simulink model "SIM_model_model_befMERGE"  (R2026a)
settings: Solver=ode4  StopTime=10  FixedStep=0.01
InitFcn:
  | initFcn;
undefined symbols (not defined in the file or in its folder): rocket
libraries: aerolibasang x2, aerolibanim x1, simulink x1, aerolibfltsims x1, aerolibatmos2 x1, aerolibadyn x1
settings Model: Creator=carlos  LastModifiedBy=carlos

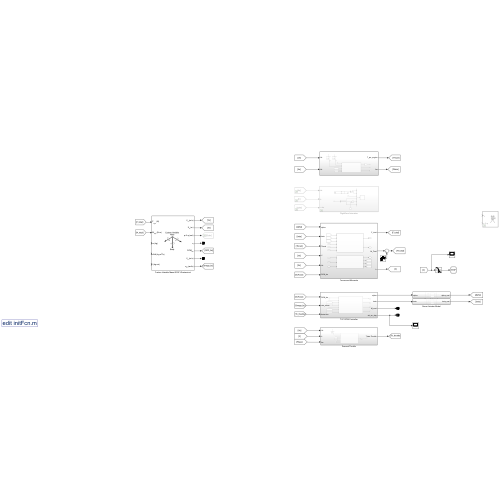
[thumbnail: Simulink's stored preview of the top-level diagram]
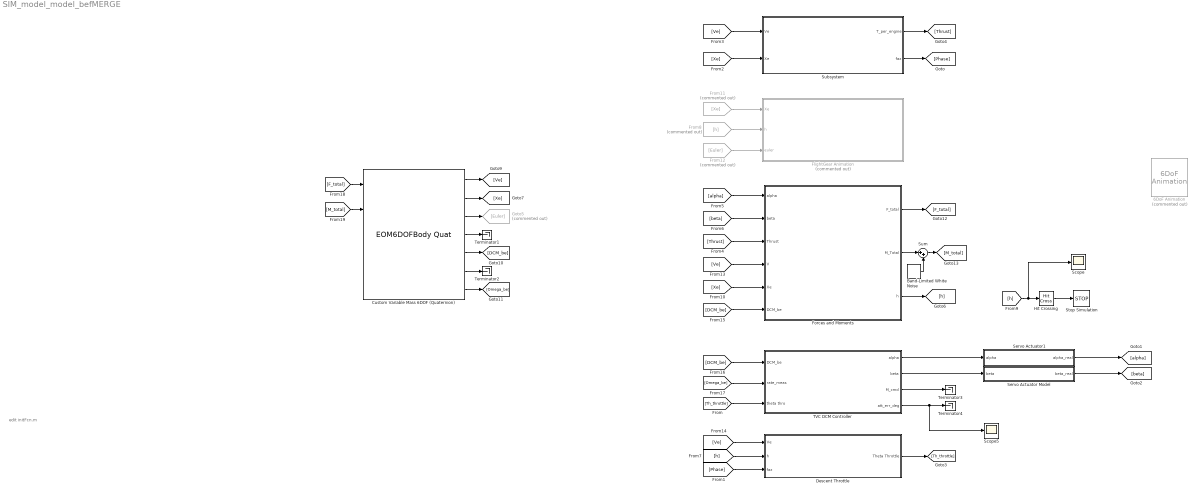
== system SIM_model_model_befMERGE ==
  note: edit initFcn.m
  6DoF Animation : aerolibanim/6DoF Animation  Commented=on  u1=[-100 100 -100 100 0 3000]  u2=0.1  u3=200  u4=[0 0 0]  u5=Fixed position  u6=[7500 7500 -3150]  u7=10  u8=on
  Band-Limited White Noise : simulink/Sources/Band-Limited White Noise  Cov=4e-6  Ts=0.01  seed=[23341 23342 23343]
  Custom Variable Mass 6DOF (Quaternion) : EOM6DOFBodyQuat  mtype=Custom Variable  eul_0=[0 deg2rad(90) 0]
  Descent Throttle : Subsystem
  FlightGear Animation : Subsystem  Commented=on
  Forces and Moments : Subsystem
  From11 : From  Commented=on  GotoTag=Xe
  From12 : From  Commented=on  GotoTag=Euler
  From8 : From  Commented=on  GotoTag=h
  Goto5 : Goto  Commented=on  GotoTag=Euler
  Hit Crossing : HitCross  HitCrossingDirection=falling
  Scope : Scope
      settings: ActiveDisplayYMinimum=-1.94208  ActiveDisplayYMaximum=17.47869
  Scope5 : Scope
      settings: ActiveDisplayYMinimum=-20.36974  ActiveDisplayYMaximum=7.70273  DataLoggingVariableName=ScopeData7
  Servo Actuator Model : Subsystem
  Servo Actuator1 : Subsystem
  Stop Simulation : Stop
  Subsystem : Subsystem
  Sum : Sum  Inputs=|++
  TVC DCM Controller : Subsystem
  Terminator{1..4} (4 alike) : Terminator
  wires:
  Sum/1 -> [M_total]
  Forces and Moments/2(M_Total) -> Sum/1
  Band-Limited White Noise/1 -> Sum/2
  [alpha] -> Forces and Moments/1(alpha)
  [DCM_be] -> Forces and Moments/6(DCM_be)
  [beta] -> Forces and Moments/2(beta)
  [Xe] -> Forces and Moments/5(Xe)
  [Thrust] -> Forces and Moments/3(Thrust)
  Forces and Moments/3(h) -> [h]
  Forces and Moments/1(F_total) -> [F_total]
  [Ve] -> Forces and Moments/4(V)
  Custom Variable Mass 6DOF (Quaternion)/1 -> [Ve]
  Custom Variable Mass 6DOF (Quaternion)/2 -> [Xe]
  Custom Variable Mass 6DOF (Quaternion)/5 -> [DCM_be]
  Custom Variable Mass 6DOF (Quaternion)/7 -> [Omega_be]
  Custom Variable Mass 6DOF (Quaternion)/6 -> Terminator2/1
  Custom Variable Mass 6DOF (Quaternion)/4 -> Terminator1/1
  [M_total] -> Custom Variable Mass 6DOF (Quaternion)/2
  [F_total] -> Custom Variable Mass 6DOF (Quaternion)/1
  Custom Variable Mass 6DOF (Quaternion)/3 -> Goto5/1
  [h] -> Descent Throttle/2(h)
  TVC DCM Controller/4(att_err_deg) -> Scope5/1, Terminator4/1
  [DCM_be] -> TVC DCM Controller/1(DCM_be)
  [Th_throttle] -> TVC DCM Controller/3(theta thro)
  [Phase] -> Descent Throttle/3(faz)
  [Omega_be] -> TVC DCM Controller/2(rate_meas)
  Descent Throttle/1(Theta Throttle) -> [Th_throttle]
  [Ve] -> Descent Throttle/1(Ve)
  Servo Actuator1/1(alpha_real) -> [alpha]
  TVC DCM Controller/3(M_cmd) -> Terminator3/1
  TVC DCM Controller/2(beta) -> Servo Actuator Model/1(beta)
  Servo Actuator Model/1(beta_real) -> [beta]
  TVC DCM Controller/1(alpha) -> Servo Actuator1/1(alpha)
  Subsystem/2(faz) -> [Phase]
  Subsystem/1(T_per_engine) -> [Thrust]
  [Ve] -> Subsystem/1(Ve)
  [Xe] -> Subsystem/2(Xe)
  From8/1 -> FlightGear Animation/2(h)
  From12/1 -> FlightGear Animation/3(euler)
  From11/1 -> FlightGear Animation/1(Xe)
  [h] -> Scope/1, Hit Crossing/1
  Hit Crossing/1 -> Stop Simulation/1

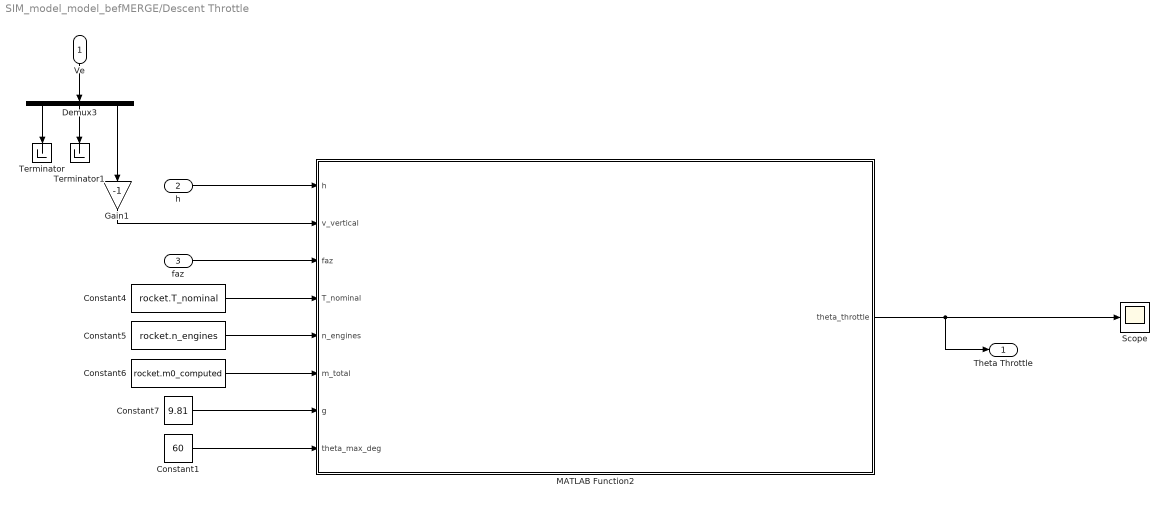
== system SIM_model_model_befMERGE/Descent Throttle ==
  Ve : Inport
  h : Inport  Port=2
  faz : Inport  Port=3
  Constant1 : Constant  Value=60
  Constant4 : Constant  Value=rocket.T_nominal
  Constant5 : Constant  Value=rocket.n_engines
  Constant6 : Constant  Value=rocket.m0_computed
  Constant7 : Constant  Value=9.81
  Demux3 : Demux  Outputs=3
  Gain1 : Gain  Gain=-1
  MATLAB Function2 : MATLAB Function  TreatAsAtomicUnit=on
  Scope : Scope
      settings: ActiveDisplayYMinimum=-0.1309  ActiveDisplayYMaximum=1.1781  DataLoggingVariableName=ScopeData6
  Terminator : Terminator
  Terminator1 : Terminator
  Theta Throttle : Outport
  wires:
  Ve/1 -> Demux3/1
  Demux3/3 -> Gain1/1
  Demux3/2 -> Terminator1/1
  Demux3/1 -> Terminator/1
  h/1 -> MATLAB Function2/1(h)
  Gain1/1 -> MATLAB Function2/2(v_vertical)
  Constant7/1 -> MATLAB Function2/7(g)
  Constant5/1 -> MATLAB Function2/5(n_engines)
  Constant6/1 -> MATLAB Function2/6(m_total)
  Constant4/1 -> MATLAB Function2/4(T_nominal)
  MATLAB Function2/1(theta_throttle) -> Theta Throttle/1, Scope/1
  faz/1 -> MATLAB Function2/3(faz)
  Constant1/1 -> MATLAB Function2/8(theta_max_deg)

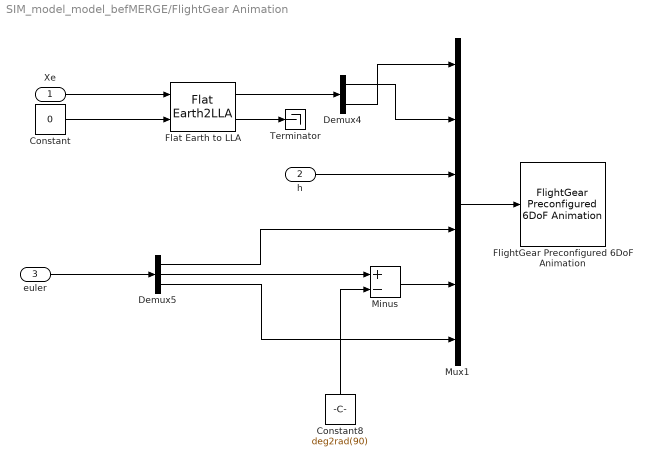
== system SIM_model_model_befMERGE/FlightGear Animation ==
  Xe : Inport
  h : Inport  Port=2
  euler : Inport  Port=3
  Constant : Constant  Value=0
  Constant8 : Constant  Value=deg2rad(90)
  Demux4 : Demux  Outputs=2
  Demux5 : Demux  Outputs=3
  Flat Earth to LLA : FlatEarth2LLA  R=6378137  LL0=[37.61889 -122.37500]
  FlightGear Preconfigured 6DoF Animation : aerolibfltsims/FlightGear Preconfigured 6DoF Animation  xFlightGearVersion=v2019.1  DestinationIpAddress=127.0.0.1  DestinationPort=5502  SampleTime=1/30  packetVersion=24
  Minus : Sum  Inputs=+-
  Mux1 : Mux  Inputs=6
  Terminator : Terminator
  wires:
  Constant/1 -> Flat Earth to LLA/2
  Demux4/1 -> Mux1/2
  Constant8/1 -> Minus/2
  Demux5/2 -> Minus/1
  Minus/1 -> Mux1/5
  Demux5/1 -> Mux1/4
  Demux5/3 -> Mux1/6
  Mux1/1 -> FlightGear Preconfigured 6DoF Animation/1
  Demux4/2 -> Mux1/1
  Flat Earth to LLA/1 -> Demux4/1
  Flat Earth to LLA/2 -> Terminator/1
  euler/1 -> Demux5/1
  h/1 -> Mux1/3
  Xe/1 -> Flat Earth to LLA/1

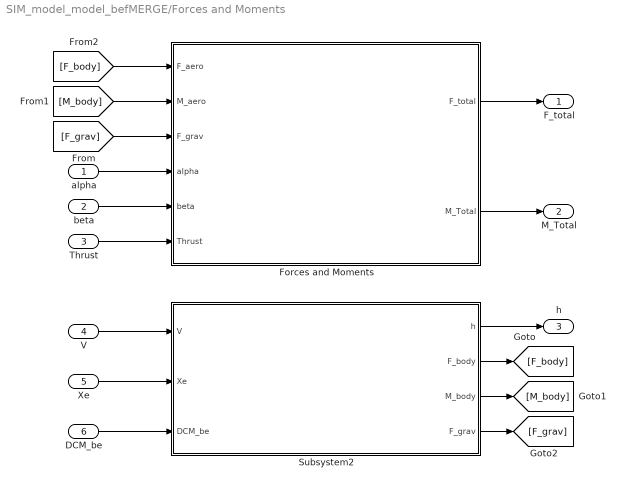
== system SIM_model_model_befMERGE/Forces and Moments ==
  alpha : Inport
  beta : Inport  Port=2
  Thrust : Inport  Port=3
  V : Inport  Port=4
  Xe : Inport  Port=5
  DCM_be : Inport  Port=6
  Forces and Moments : Subsystem
  Subsystem2 : Subsystem
  F_total : Outport
  M_Total : Outport  Port=2
  h : Outport  Port=3
  wires:
  alpha/1 -> Forces and Moments/4(alpha)
  DCM_be/1 -> Subsystem2/3(DCM_be)
  Xe/1 -> Subsystem2/2(Xe)
  beta/1 -> Forces and Moments/5(beta)
  Thrust/1 -> Forces and Moments/6(Thrust)
  Forces and Moments/2(M_Total) -> M_Total/1
  Forces and Moments/1(F_total) -> F_total/1
  Subsystem2/1(h) -> h/1
  V/1 -> Subsystem2/1(V)
  [F_grav] -> Forces and Moments/3(F_grav)
  [M_body] -> Forces and Moments/2(M_aero)
  [F_body] -> Forces and Moments/1(F_aero)
  Subsystem2/2(F_body) -> [F_body]
  Subsystem2/4(F_grav) -> [F_grav]
  Subsystem2/3(M_body) -> [M_body]

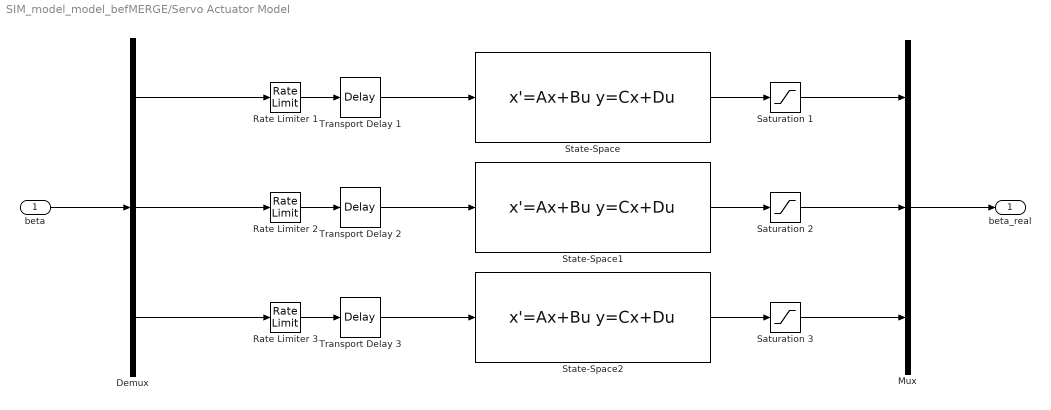
== system SIM_model_model_befMERGE/Servo Actuator Model ==
  beta : Inport
  Demux : Demux  Outputs=3
  Mux : Mux  Inputs=3
  Rate Limiter 1 : RateLimiter  RisingSlewLimit=deg2rad(rocket.servo.max_rate_dps)  FallingSlewLimit=-deg2rad(rocket.servo.max_rate_dps)  SampleTimeMode=inherited
  Rate Limiter 2 : RateLimiter  RisingSlewLimit=deg2rad(rocket.servo.max_rate_dps)  FallingSlewLimit=-deg2rad(rocket.servo.max_rate_dps)  SampleTimeMode=inherited
  Rate Limiter 3 : RateLimiter  RisingSlewLimit=deg2rad(rocket.servo.max_rate_dps)  FallingSlewLimit=-deg2rad(rocket.servo.max_rate_dps)  SampleTimeMode=inherited
  Saturation 1 : Saturate  UpperLimit=deg2rad(75)  LowerLimit=deg2rad(-75)
  Saturation 2 : Saturate  UpperLimit=deg2rad(75)  LowerLimit=deg2rad(-75)
  Saturation 3 : Saturate  UpperLimit=deg2rad(75)  LowerLimit=deg2rad(-75)
  State-Space : StateSpace  A="[0  1; -rocket.servo.wn^2  -2*rocket.servo.zeta*rocket.servo.wn]"  B=[0; rocket.servo.wn^2]  C="[1  0]"  D=0  InitialCondition=[0;0]
  State-Space1 : StateSpace  A="[0  1; -rocket.servo.wn^2  -2*rocket.servo.zeta*rocket.servo.wn]"  B=[0; rocket.servo.wn^2]  C="[1  0]"  D=0  InitialCondition=[0;0]
  State-Space2 : StateSpace  A="[0  1; -rocket.servo.wn^2  -2*rocket.servo.zeta*rocket.servo.wn]"  B=[0; rocket.servo.wn^2]  C="[1  0]"  D=0  InitialCondition=[0;0]
  Transport Delay 1 : TransportDelay  DelayTime=rocket.servo.delay_s
  Transport Delay 2 : TransportDelay  DelayTime=rocket.servo.delay_s
  Transport Delay 3 : TransportDelay  DelayTime=rocket.servo.delay_s
  beta_real : Outport
  wires:
  Saturation 2/1 -> Mux/2
  beta/1 -> Demux/1
  State-Space1/1 -> Saturation 2/1
  Transport Delay 2/1 -> State-Space1/1
  Saturation 1/1 -> Mux/1
  Saturation 3/1 -> Mux/3
  Mux/1 -> beta_real/1
  Rate Limiter 2/1 -> Transport Delay 2/1
  Transport Delay 1/1 -> State-Space/1
  Demux/3 -> Rate Limiter 3/1
  Demux/1 -> Rate Limiter 1/1
  Demux/2 -> Rate Limiter 2/1
  Rate Limiter 3/1 -> Transport Delay 3/1
  State-Space2/1 -> Saturation 3/1
  Transport Delay 3/1 -> State-Space2/1
  State-Space/1 -> Saturation 1/1
  Rate Limiter 1/1 -> Transport Delay 1/1

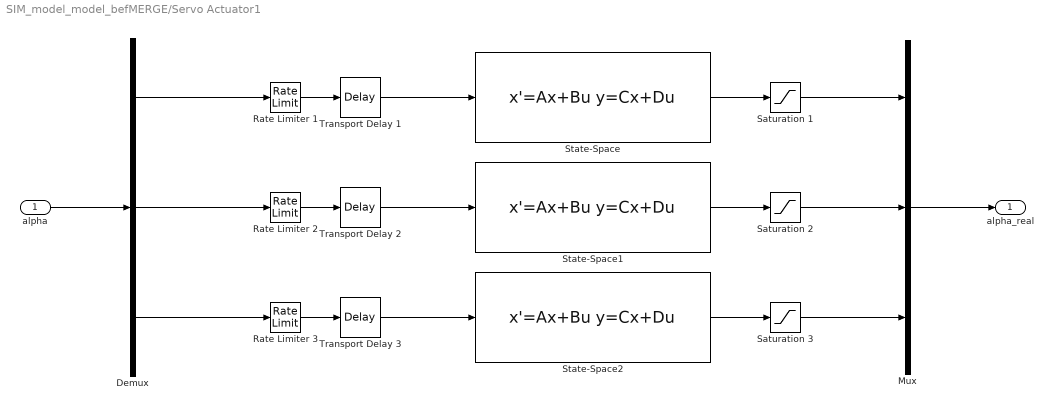
== system SIM_model_model_befMERGE/Servo Actuator1 ==
  alpha : Inport
  Demux : Demux  Outputs=3
  Mux : Mux  Inputs=3
  Rate Limiter 1 : RateLimiter  RisingSlewLimit=deg2rad(rocket.servo.max_rate_dps)  FallingSlewLimit=-deg2rad(rocket.servo.max_rate_dps)  SampleTimeMode=inherited
  Rate Limiter 2 : RateLimiter  RisingSlewLimit=deg2rad(rocket.servo.max_rate_dps)  FallingSlewLimit=-deg2rad(rocket.servo.max_rate_dps)  SampleTimeMode=inherited
  Rate Limiter 3 : RateLimiter  RisingSlewLimit=deg2rad(rocket.servo.max_rate_dps)  FallingSlewLimit=-deg2rad(rocket.servo.max_rate_dps)  SampleTimeMode=inherited
  Saturation 1 : Saturate  UpperLimit=deg2rad(75)  LowerLimit=deg2rad(-75)
  Saturation 2 : Saturate  UpperLimit=deg2rad(75)  LowerLimit=deg2rad(-75)
  Saturation 3 : Saturate  UpperLimit=deg2rad(75)  LowerLimit=deg2rad(-75)
  State-Space : StateSpace  A="[0  1; -rocket.servo.wn^2  -2*rocket.servo.zeta*rocket.servo.wn]"  B=[0; rocket.servo.wn^2]  C="[1  0]"  D=0  InitialCondition=[0;0]
  State-Space1 : StateSpace  A="[0  1; -rocket.servo.wn^2  -2*rocket.servo.zeta*rocket.servo.wn]"  B=[0; rocket.servo.wn^2]  C="[1  0]"  D=0  InitialCondition=[0;0]
  State-Space2 : StateSpace  A="[0  1; -rocket.servo.wn^2  -2*rocket.servo.zeta*rocket.servo.wn]"  B=[0; rocket.servo.wn^2]  C="[1  0]"  D=0  InitialCondition=[0;0]
  Transport Delay 1 : TransportDelay  DelayTime=rocket.servo.delay_s
  Transport Delay 2 : TransportDelay  DelayTime=rocket.servo.delay_s
  Transport Delay 3 : TransportDelay  DelayTime=rocket.servo.delay_s
  alpha_real : Outport
  wires:
  Rate Limiter 1/1 -> Transport Delay 1/1
  State-Space/1 -> Saturation 1/1
  Transport Delay 1/1 -> State-Space/1
  alpha/1 -> Demux/1
  Transport Delay 2/1 -> State-Space1/1
  State-Space1/1 -> Saturation 2/1
  Rate Limiter 2/1 -> Transport Delay 2/1
  Rate Limiter 3/1 -> Transport Delay 3/1
  State-Space2/1 -> Saturation 3/1
  Transport Delay 3/1 -> State-Space2/1
  Demux/3 -> Rate Limiter 3/1
  Demux/2 -> Rate Limiter 2/1
  Demux/1 -> Rate Limiter 1/1
  Saturation 1/1 -> Mux/1
  Saturation 2/1 -> Mux/2
  Saturation 3/1 -> Mux/3
  Mux/1 -> alpha_real/1

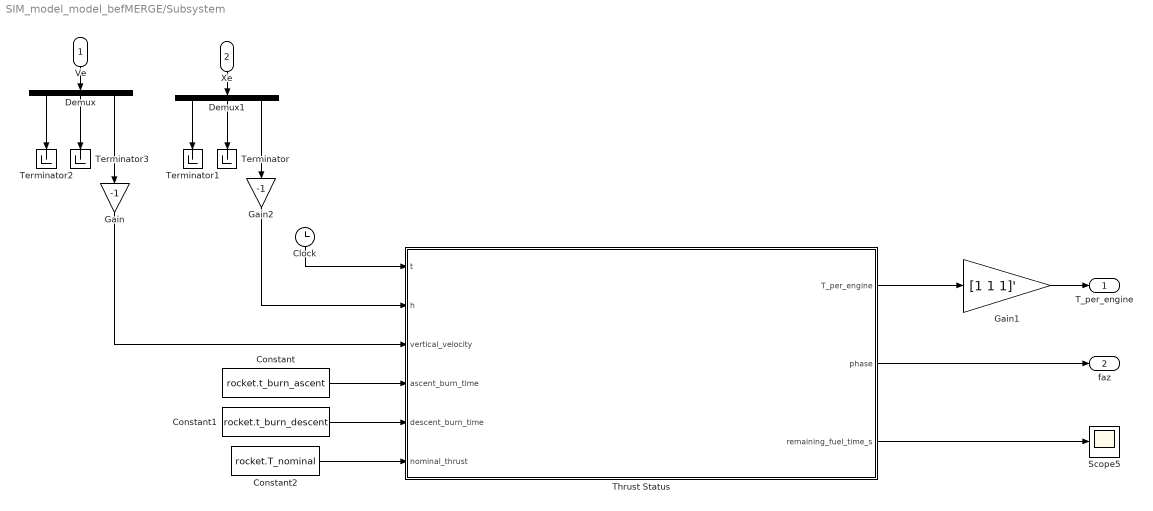
== system SIM_model_model_befMERGE/Subsystem ==
  Ve : Inport
  Xe : Inport  Port=2
  Clock : Clock
  Constant : Constant  Value=rocket.t_burn_ascent
  Constant1 : Constant  Value=rocket.t_burn_descent
  Constant2 : Constant  Value=rocket.T_nominal
  Demux : Demux  Outputs=3
  Demux1 : Demux  Outputs=3
  Gain : Gain  Gain=-1
  Gain1 : Gain  Gain=[1 1 1]'
  Gain2 : Gain  Gain=-1
  Scope5 : Scope
      settings: ActiveDisplayYMinimum=-1.25  ActiveDisplayYMaximum=11.25
  Terminator{,1..3} (4 alike) : Terminator
  Thrust Status : MATLAB Function  TreatAsAtomicUnit=on
  T_per_engine : Outport
  faz : Outport  Port=2
  wires:
  Ve/1 -> Demux/1
  Xe/1 -> Demux1/1
  Demux/2 -> Terminator3/1
  Thrust Status/2(phase) -> faz/1
  Demux1/3 -> Gain2/1
  Demux1/1 -> Terminator1/1
  Demux/3 -> Gain/1
  Thrust Status/3(remaining_fuel_time_s) -> Scope5/1
  Gain2/1 -> Thrust Status/2(h)
  Demux/1 -> Terminator2/1
  Demux1/2 -> Terminator/1
  Clock/1 -> Thrust Status/1(t)
  Gain/1 -> Thrust Status/3(vertical_velocity)
  Constant/1 -> Thrust Status/4(ascent_burn_time)
  Constant1/1 -> Thrust Status/5(descent_burn_time)
  Gain1/1 -> T_per_engine/1
  Constant2/1 -> Thrust Status/6(nominal_thrust)
  Thrust Status/1(T_per_engine) -> Gain1/1

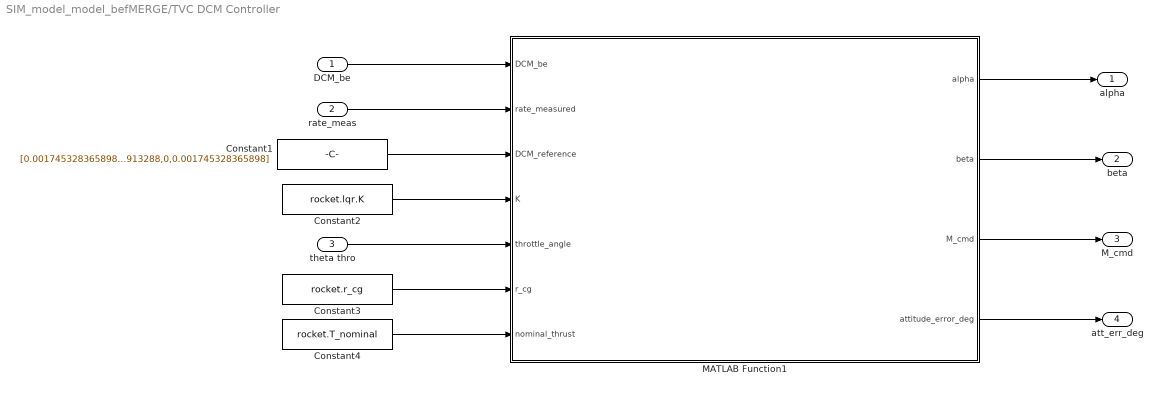
== system SIM_model_model_befMERGE/TVC DCM Controller ==
  DCM_be : Inport
  rate_meas : Inport  Port=2
  theta thro : Inport  Port=3
  Constant1 : Constant  Value=[0.001745328365898,0,-0.999998476913288;0,1,0;0.999998476913288,0,0.001745328365898]
  Constant2 : Constant  Value=rocket.lqr.K
  Constant3 : Constant  Value=rocket.r_cg
  Constant4 : Constant  Value=rocket.T_nominal
  MATLAB Function1 : MATLAB Function  TreatAsAtomicUnit=on
  alpha : Outport
  beta : Outport  Port=2
  M_cmd : Outport  Port=3
  att_err_deg : Outport  Port=4
  wires:
  Constant2/1 -> MATLAB Function1/4(K)
  rate_meas/1 -> MATLAB Function1/2(rate_measured)
  Constant1/1 -> MATLAB Function1/3(DCM_reference)
  MATLAB Function1/1(alpha) -> alpha/1
  DCM_be/1 -> MATLAB Function1/1(DCM_be)
  MATLAB Function1/2(beta) -> beta/1
  MATLAB Function1/3(M_cmd) -> M_cmd/1
  MATLAB Function1/4(attitude_error_deg) -> att_err_deg/1
  Constant3/1 -> MATLAB Function1/6(r_cg)
  Constant4/1 -> MATLAB Function1/7(nominal_thrust)
  theta thro/1 -> MATLAB Function1/5(throttle_angle)

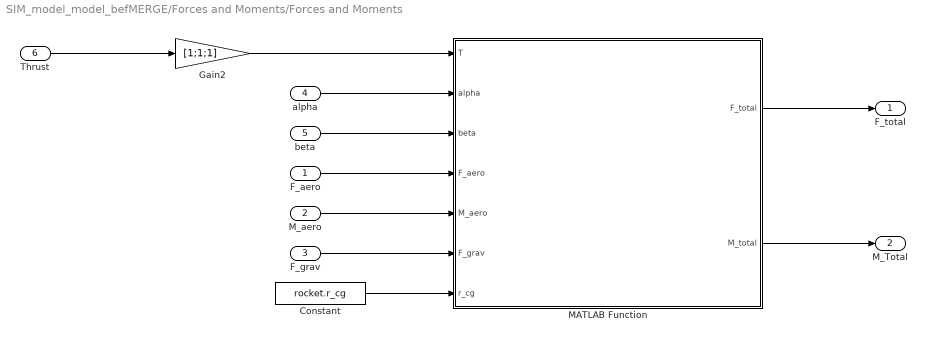
== system SIM_model_model_befMERGE/Forces and Moments/Forces and Moments ==
  F_aero : Inport
  M_aero : Inport  Port=2
  F_grav : Inport  Port=3
  alpha : Inport  Port=4
  beta : Inport  Port=5
  Thrust : Inport  Port=6
  Constant : Constant  Value=rocket.r_cg
  Gain2 : Gain  Gain=[1;1;1]
  MATLAB Function : MATLAB Function  TreatAsAtomicUnit=on
  F_total : Outport
  M_Total : Outport  Port=2
  wires:
  M_aero/1 -> MATLAB Function/5(M_aero)
  F_grav/1 -> MATLAB Function/6(F_grav)
  MATLAB Function/1(F_total) -> F_total/1
  Gain2/1 -> MATLAB Function/1(T)
  MATLAB Function/2(M_total) -> M_Total/1
  F_aero/1 -> MATLAB Function/4(F_aero)
  beta/1 -> MATLAB Function/3(beta)
  alpha/1 -> MATLAB Function/2(alpha)
  Thrust/1 -> Gain2/1
  Constant/1 -> MATLAB Function/7(r_cg)

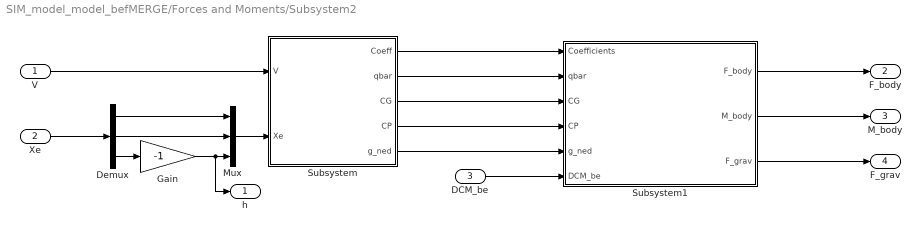
== system SIM_model_model_befMERGE/Forces and Moments/Subsystem2 ==
  V : Inport
  Xe : Inport  Port=2
  DCM_be : Inport  Port=3
  Demux : Demux  Outputs=3
  Gain : Gain  Gain=-1
  Mux : Mux  Inputs=3
  Subsystem : Subsystem
  Subsystem1 : Subsystem
  h : Outport
  F_body : Outport  Port=2
  M_body : Outport  Port=3
  F_grav : Outport  Port=4
  wires:
  Subsystem/1(Coeff) -> Subsystem1/1(Coefficients)
  Demux/1 -> Mux/1
  Demux/3 -> Gain/1
  Subsystem/3(CG) -> Subsystem1/3(CG)
  Subsystem/4(CP) -> Subsystem1/4(CP)
  Subsystem/2(qbar) -> Subsystem1/2(qbar)
  Demux/2 -> Mux/2
  Mux/1 -> Subsystem/2(Xe)
  Subsystem1/2(M_body) -> M_body/1
  Subsystem/5(g_ned) -> Subsystem1/5(g_ned)
  DCM_be/1 -> Subsystem1/6(DCM_be)
  Xe/1 -> Demux/1
  Gain/1 -> Mux/3, h/1
  V/1 -> Subsystem/1(V)
  Subsystem1/1(F_body) -> F_body/1
  Subsystem1/3(F_grav) -> F_grav/1

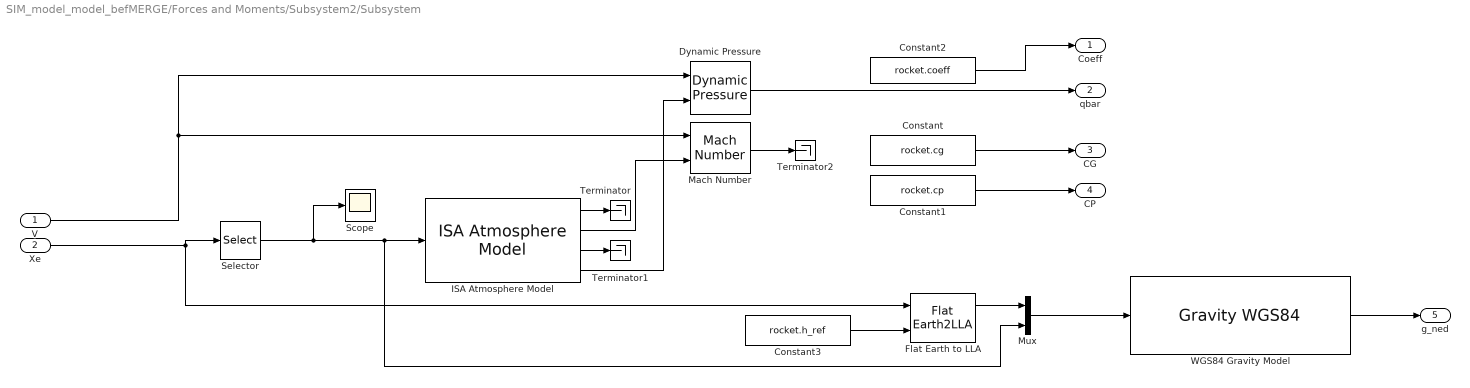
== system SIM_model_model_befMERGE/Forces and Moments/Subsystem2/Subsystem ==
  V : Inport
  Xe : Inport  Port=2
  Constant : Constant  Value=rocket.cg
  Constant1 : Constant  Value=rocket.cp
  Constant2 : Constant  Value=rocket.coeff
  Constant3 : Constant  Value=rocket.h_ref
  Dynamic Pressure : aerolibasang/Dynamic Pressure
  Flat Earth to LLA : FlatEarth2LLA  R=6378137
  ISA Atmosphere Model : aerolibatmos2/ISA Atmosphere Model  useExtended=off  action=Warning  custom=off  viscosityOut=off  g=9.80665  gamma=1.4  R=287.0531  L=0.0065  h_trop=11000  h_strat=20000  rho0=1.225  P0=101325  T0=288.15  h0=0  S=110.4  Tref=273.15  muref=1.716e-5
  Mach Number : aerolibasang/Mach Number
  Mux : Mux  Inputs=2
  Scope : Scope
      settings: ActiveDisplayYMinimum=-14.46754  ActiveDisplayYMaximum=130.20784  DataLoggingVariableName=ScopeData6
  Selector : Selector  InputPortWidth=3  IndexOptions=Index vector (dialog)  Indices=3  OutputSizes=1
  Terminator : Terminator
  Terminator1 : Terminator
  Terminator2 : Terminator
  "WGS84 Gravity Model  " : GravityWGS84
  Coeff : Outport
  qbar : Outport  Port=2
  CG : Outport  Port=3
  CP : Outport  Port=4
  g_ned : Outport  Port=5
  wires:
  V/1 -> Mach Number/1, Dynamic Pressure/1
  Mach Number/1 -> Terminator2/1
  ISA Atmosphere Model/1 -> Terminator/1
  ISA Atmosphere Model/3 -> Terminator1/1
  Xe/1 -> Selector/1, Flat Earth to LLA/1
  ISA Atmosphere Model/4 -> Dynamic Pressure/2
  ISA Atmosphere Model/2 -> Mach Number/2
  Selector/1 -> Scope/1, Mux/2, ISA Atmosphere Model/1
  Mux/1 -> "WGS84 Gravity Model  "/1
  Flat Earth to LLA/1 -> Mux/1
  Constant3/1 -> Flat Earth to LLA/2
  "WGS84 Gravity Model  "/1 -> g_ned/1
  Dynamic Pressure/1 -> qbar/1
  Constant1/1 -> CP/1
  Constant2/1 -> Coeff/1
  Constant/1 -> CG/1

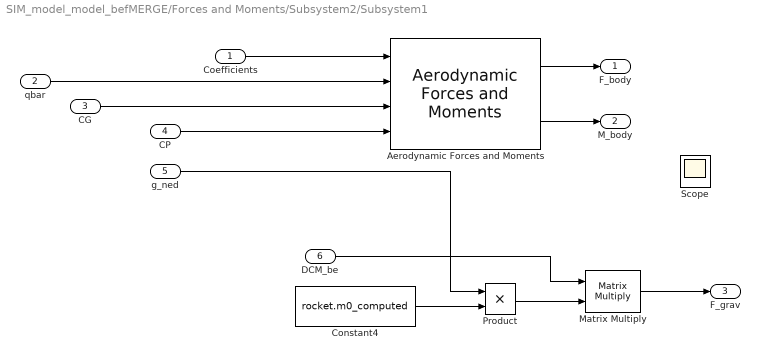
== system SIM_model_model_befMERGE/Forces and Moments/Subsystem2/Subsystem1 ==
  Coefficients : Inport
  qbar : Inport  Port=2
  CG : Inport  Port=3
  CP : Inport  Port=4
  g_ned : Inport  Port=5
  DCM_be : Inport  Port=6
  "Aerodynamic Forces and Moments " : aerolibadyn/Aerodynamic Forces and Moments   inputAxes=Body  outputForceAxes=Body  outputMomentAxes=Body  S=0.0854  b=0.0742  cbar=1.15
  Constant4 : Constant  Value=rocket.m0_computed
  Matrix Multiply : Product  Multiplication=Matrix(*)
  Product : Product
  Scope : Scope
      settings: ActiveDisplayYMinimum=-1  ActiveDisplayYMaximum=1  DataLoggingVariableName=ScopeData4
  F_body : Outport
  M_body : Outport  Port=2
  F_grav : Outport  Port=3
  wires:
  g_ned/1 -> Product/1
  qbar/1 -> "Aerodynamic Forces and Moments "/2
  Coefficients/1 -> "Aerodynamic Forces and Moments "/1
  "Aerodynamic Forces and Moments "/1 -> F_body/1
  Matrix Multiply/1 -> F_grav/1
  CG/1 -> "Aerodynamic Forces and Moments "/3
  "Aerodynamic Forces and Moments "/2 -> M_body/1
  Constant4/1 -> Product/2
  DCM_be/1 -> Matrix Multiply/1
  CP/1 -> "Aerodynamic Forces and Moments "/4
  Product/1 -> Matrix Multiply/2

== matlab function SIM_model_model_befMERGE/Descent Throttle/MATLAB Function2 ==
  settings: updateMethod=DISCRETE
  data: theta_throttle output; h input; v_vertical input; faz input; T_nominal input; n_engines input; m_total input; g input; theta_max_deg input
function theta_throttle = descent_tilt_lqr(h, v_vertical, faz, T_nominal, n_engines, m_total, g, theta_max_deg)
    if faz ~= 3
        theta_throttle = 0;
        return;
    end

    T_max_toplam = n_engines * T_nominal;
    theta_max = deg2rad(theta_max_deg);

    theta_hover = acos(min(max(m_total*g/T_max_toplam, -1), 1));

    K_H = -0.2;
    K_V = -0.37986389;

    delta_theta = -(K_H*h + K_V*v_vertical);
    theta_throttle = theta_hover + delta_theta;

    theta_throttle = min(max(theta_throttle, 0), theta_max);

end

== matlab function SIM_model_model_befMERGE/Forces and Moments/Forces and Moments/MATLAB Function ==
  data: T input; F_total output; alpha input; beta input; F_aero input; M_aero input; F_grav input; M_total output; r_cg input
function [F_total, M_total] = rocket_forces_moments(T, alpha, beta, F_aero, M_aero, F_grav, r_cg)

    F_thrust = zeros(3,1);
    M_thrust = zeros(3,1);

    for i = 1:3
        F_i = T(i) * [cos(alpha(i))*cos(beta(i));
                       sin(alpha(i))*cos(beta(i));
                       sin(beta(i))];

        r_i = r_cg(:,i);
        M_i = cross(r_i, F_i);

        F_thrust = F_thrust + F_i;
        M_thrust = M_thrust + M_i;
    end

    F_total = F_thrust + F_aero + F_grav;
    M_total = M_thrust + M_aero;

end

== matlab function SIM_model_model_befMERGE/TVC DCM Controller/MATLAB Function1 ==
  settings: updateMethod=DISCRETE
  data: DCM_be input; alpha output; rate_measured input; DCM_reference input; K input; beta output; M_cmd output; throttle_angle input; attitude_error_deg output; r_cg input; nominal_thrust input
function [alpha, beta, M_cmd, attitude_error_deg] = ...
    tvc_controller_dcm(DCM_be, rate_measured, DCM_reference, ...
                       K, throttle_angle, r_cg, nominal_thrust)

    DCM_be        = reshape(DCM_be,        3, 3);
    DCM_reference = reshape(DCM_reference, 3, 3);
    r_cg          = reshape(r_cg,          3, 3);

    gimbal_limit_rad = deg2rad([-10, 10]);

    gimbal_min = gimbal_limit_rad(1);
    gimbal_max = gimbal_limit_rad(2);

    DCM_error = DCM_be * DCM_reference';

    attitude_error = 0.5 * ...
        [DCM_error(3,2) - DCM_error(2,3);
         DCM_error(1,3) - DCM_error(3,1);
         DCM_error(2,1) - DCM_error(1,2)];

    state_error = [attitude_error;
                   rate_measured];

    M_cmd = -K * state_error;

    attitude_error_deg = rad2deg(attitude_error);

    allocation_matrix = zeros(3,6);

    for i = 1:3
        r_i = r_cg(:,i);

        allocation_matrix(:, 2*i-1) = ...
            cross(r_i, nominal_thrust * [0; 1; 0]);

        allocation_matrix(:, 2*i) = ...
            cross(r_i, nominal_thrust * [0; 0; 1]);
    end

    delta_lqr = pinv(allocation_matrix) * M_cmd;

    max_gimbal_command = max(abs(delta_lqr));

    if max_gimbal_command > gimbal_max
        delta_lqr = delta_lqr * ...
            (gimbal_max / max_gimbal_command);
    end

    alpha = zeros(3,1);
    beta  = zeros(3,1);

    for i = 1:3

        azimuth_angle = atan2(r_cg(3,i), r_cg(2,i));

        alpha_nominal = atan2( ...
            sin(throttle_angle) * cos(azimuth_angle), ...
            cos(throttle_angle));

        beta_nominal = asin( ...
            sin(throttle_angle) * sin(azimuth_angle));

        alpha(i) = alpha_nominal + delta_lqr(2*i-1);
        beta(i)  = beta_nominal  + delta_lqr(2*i);

    end

    overall_gimbal_limit = max( ...
        abs(gimbal_max), ...
        throttle_angle + gimbal_max);

    alpha = min( ...
        max(alpha, -overall_gimbal_limit), ...
        overall_gimbal_limit);

    beta = min( ...
        max(beta, -overall_gimbal_limit), ...
        overall_gimbal_limit);

end

== matlab function SIM_model_model_befMERGE/Subsystem/Thrust Status ==
  settings: updateMethod=DISCRETE
  data: t input; h input; T_per_engine output; vertical_velocity input; ascent_burn_time input; descent_burn_time input; nominal_thrust input; phase output; remaining_fuel_time_s output
function [T_per_engine, phase, remaining_fuel_time_s] = ...
    engine_thrust_status(t, h, vertical_velocity, ...
                        ascent_burn_time, descent_burn_time, nominal_thrust)

    ignition_altitude_m = 15;

    persistent phase_state ignition_time

    if isempty(phase_state)
        phase_state = int8(1);
        ignition_time = 0;
    end

    if phase_state == 1

        if t < ascent_burn_time
            T_per_engine = nominal_thrust;
        else
            phase_state = int8(2);
            T_per_engine = 0;
        end

        remaining_fuel_time_s = descent_burn_time;

    elseif phase_state == 2

        T_per_engine = 0;

        if vertical_velocity < 0 && h <= ignition_altitude_m
            phase_state = int8(3);
            ignition_time = t;
        end

        remaining_fuel_time_s = descent_burn_time;

    else

        elapsed_time = t - ignition_time;

        remaining_fuel_time_s = max( ...
            descent_burn_time - elapsed_time, 0);

        if remaining_fuel_time_s <= 0
            phase_state = int8(4);
            T_per_engine = 0;
        else
            T_per_engine = nominal_thrust;
        end

    end

    phase = double(phase_state);

end
